simulink model "Calibration_250328"  (R2024b)
settings: Solver=VariableStepAuto  StartTime=0.0  StopTime=Sim.Cal_EndTime  RelTol=1e-3
values from neighbouring files (symbols this model uses):
  m = obj.Br *obj.volume / obj.mu    [External_Magnet2.m]
  Sim = Call_MagneticBasket_Params    [Test.m]    (also in execute_calibrated_result.m; execute_optimized_result.m; optimize_for_calibration.m; optimize_for_max_bending.m)
undefined symbols (not defined in the file or in its folder): X, Y, Z
libraries: sm_lib x64, nesl_utility x43, matrix_library x18, vrlib x12
(part 2 of 2)

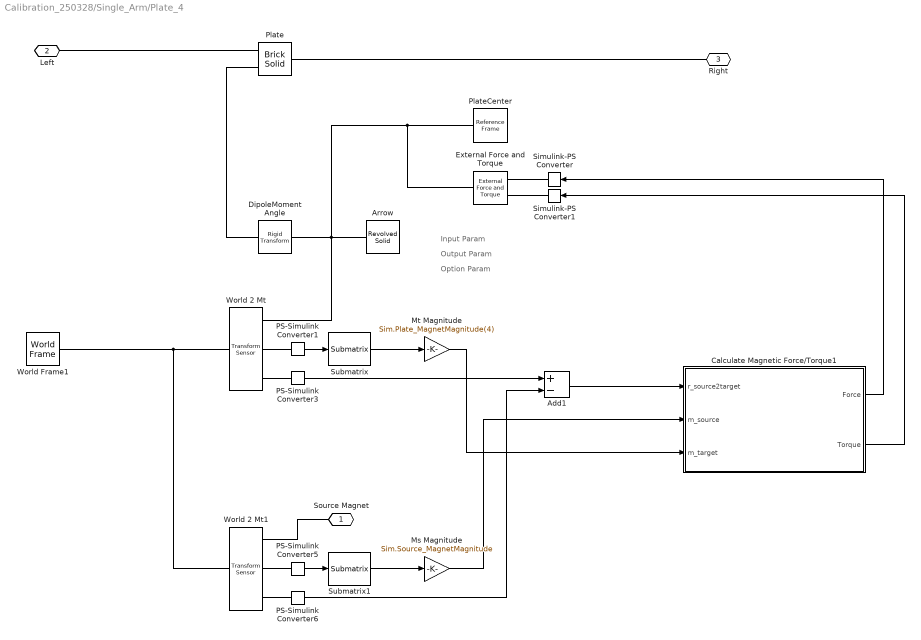
== system Calibration_250328/Single_Arm/Plate_4 ==
  note: Input Param
  note: Output Param
  note: Option Param
  Add1 : Sum  Inputs=+-
  Arrow : sm_lib/Body Elements/Revolved Solid  RevolutionCrossSection=[0 20; 0 0; 1 0; 1 15; 2 15]/10  RevolutionCrossSectionUnits=mm  RevolutionExtent=Full  RevolutionAngle=180  RevolutionAngleUnits=deg  ExportConvexHullGeometry=off  InertiaType=CalculateFromGeometry  BasedOnType=Density  Density=0  DensityUnits=kg/m^3  Mass=1  MassUnits=kg  CenterOfMass=[0 0 0]  CenterOfMassUnits=m  MomentsOfInertia=[1 1 1]  MomentsOfInertiaUnits=kg*m^2  ProductsOfInertia=[0 0 0]  ProductsOfInertiaUnits=kg*m^2  GraphicType=FromGeometry  MarkerShape=Sphere  MarkerSize=10  GraphicVisPropType=SimpleVisualProperties  GraphicDiffuseColor=[0.8 0.0 0.0]  GraphicOpacity=1  GraphicSpecularColor=[0.5 0.5 0.5 1.0]  GraphicAmbientColor=[0.15 0.15 0.15 1.0]  GraphicEmissiveColor=[0.0 0.0 0.0 1.0]  GraphicShininess=75  DoExposeReferenceFrame=on  SerializedFrames=<Frames/>
  Calculate Magnetic Force/Torque1 : Subsystem  AncestorBlock=Manget_DipoleMomentModel_Library_250306/Calculate Magnetic Force//Torque
  DipoleMoment Angle : sm_lib/Frames and Transforms/Rigid Transform  RotationMethod=StandardAxis  FollAlignAxisA=+X  BaseAlignAxisA=+Y  FollAlignAxisB=+Y  BaseAlignAxisB=+Z  RotationStandardAxis=+X  RotationAngle=Sim.Angle(4)  RotationAngleUnits=rad  RotationArbitraryAxis=[0 0 1]  RotationSequenceAxes=FollowerAxes  RotationSequence=XYX  RotationSequenceAngles=[0 0 0]  RotationSequenceAnglesUnits=deg  RotationMatrix=[1 0 0; 0 1 0; 0 0 1]  Quaternion=[1 0 0 0]  TranslationMethod=None  TranslationCartesianOffset=[0 0 0]  TranslationCartesianOffsetUnits=m  TranslationStandardAxis=+Z  TranslationStandardOffset=0  TranslationStandardOffsetUnits=m  TranslationROffset=0  TranslationROffsetUnits=m  TranslationThetaOffset=0  TranslationThetaOffsetUnits=deg  TranslationZOffset=0  TranslationZOffsetUnits=m
  External Force and Torque : sm_lib/Forces and Torques/External Force and Torque  EnableForceX=off  EnableForceY=off  EnableForceZ=off  EnableForce=on  ForceResolutionFrame=World  EnableTorqueX=off  EnableTorqueY=off  EnableTorqueZ=off  EnableTorque=on  TorqueResolutionFrame=World
  Ms Magnitude : Gain  Gain=Sim.Source_MagnetMagnitude
  Mt Magnitude : Gain  Gain=Sim.Plate_MagnetMagnitude(4)
  PS-Simulink Converter{1,3,5..6} (4 alike) : nesl_utility/PS-Simulink Converter  PhysicalDomain=network_engine_domain  SubClassName=ps_output  LeftPortType=input  RightPortType=output  PseudoPeriodic=off  Frequencies=[]  VectorFormat=inherit  Unit=inherit  AffineConversion=off
  Plate : sm_lib/Body Elements/Brick Solid  BrickDimensions=[Sim.PlateWidth Sim.PlateLength Sim.PlateThickness]  BrickDimensionsUnits=m  ExportEntireGeometry=off  InertiaType=CalculateFromGeometry  BasedOnType=Density  Density=Sim.PlateDensity  DensityUnits=kg/m^3  Mass=1  MassUnits=kg  CenterOfMass=[0 0 0]  CenterOfMassUnits=m  MomentsOfInertia=[1 1 1]  MomentsOfInertiaUnits=kg*m^2  ProductsOfInertia=[0 0 0]  ProductsOfInertiaUnits=kg*m^2  GraphicType=FromGeometry  MarkerShape=Sphere  MarkerSize=10  GraphicVisPropType=SimpleVisualProperties  GraphicDiffuseColor=[0.5 0.5 0.5]  GraphicOpacity=0.5  GraphicSpecularColor=[0.5 0.5 0.5 1.0]  GraphicAmbientColor=[0.15 0.15 0.15 1.0]  GraphicEmissiveColor=[0.0 0.0 0.0 1.0]  GraphicShininess=75  DoExposeReferenceFrame=off  SerializedFrames=<Frames><Frame><Id>Frame1</Id><Value><Name>F1</Name><Origin><Source>GeometricFeature</Source><FeatureName>-y -z curve</FeatureName></Origin><PrimaryAxis><DefinedDirection>+Z</DefinedDirection><Source>ReferenceFrame</Source><SourceDirection>+X</SourceDirection><FeatureName></FeatureName></PrimaryAxis><SecondaryAxis><DefinedDirection>+X</DefinedDirection><Source>ReferenceFrame</Source><SourceDirection>+Y</SourceDirection><FeatureName></FeatureName></SecondaryAxis></Value></Frame><Frame><Id>Frame2</Id><Value><Name>F2</Name><Origin><Source>GeometricFeature</Source><FeatureName>+y -z curve</FeatureName></Origin><PrimaryAxis><DefinedDirection>+Z</DefinedDirection><Source>ReferenceFrame</Source><SourceDirection>+X</SourceDirection><FeatureName></FeatureName></PrimaryAxis><SecondaryAxis><DefinedDirection>+X</DefinedDirection><Source>ReferenceFrame</Source><SourceDirection>+Y</SourceDirection><FeatureName></FeatureName></SecondaryAxis></Value></Frame><Frame><Id>Frame3</Id><Value><Name>F3</Name><Origin><Source>ReferenceFrame</Source><FeatureName></FeatureName></Origin><PrimaryAxis><DefinedDirection>+Z</DefinedDirection><Source>ReferenceFrame</Source><SourceDirection>+Y</SourceDirection><FeatureName></FeatureName></PrimaryAxis><SecondaryAxis><DefinedDirection>+X</DefinedDirection><Source>ReferenceFrame</Source><SourceDirection>+X</SourceDirection><FeatureName></FeatureName></SecondaryAxis></Value></Frame></Frames>
  PlateCenter : sm_lib/Frames and Transforms/Reference Frame
  Simulink-PS Converter : nesl_utility/Simulink-PS Converter  PhysicalDomain=network_engine_domain  SubClassName=ps_input  LeftPortType=input  RightPortType=output  PseudoPeriodic=off  Frequencies=[]  NoiseDistribution=none  NoiseParameters=[]  Unit=1  AffineConversion=off  FilteringAndDerivatives=filter  SimscapeFilterOrder=2  InputFilterTimeConstant=0.001  UdotUserProvided=0
  Simulink-PS Converter1 : nesl_utility/Simulink-PS Converter  PhysicalDomain=network_engine_domain  SubClassName=ps_input  LeftPortType=input  RightPortType=output  PseudoPeriodic=off  Frequencies=[]  NoiseDistribution=none  NoiseParameters=[]  Unit=1  AffineConversion=off  FilteringAndDerivatives=filter  SimscapeFilterOrder=2  InputFilterTimeConstant=0.001  UdotUserProvided=0
  Submatrix : matrix_library/Submatrix  RowSpan=All rows  RowStartMode=First  RowStartIndex=1  RowEndMode=Last  RowEndIndex=1  ColSpan=One column  ColStartMode=Last  ColStartIndex=1  ColEndMode=Last  ColEndIndex=1
  Submatrix1 : matrix_library/Submatrix  RowSpan=All rows  RowStartMode=First  RowStartIndex=1  RowEndMode=Last  RowEndIndex=1  ColSpan=One column  ColStartMode=Last  ColStartIndex=1  ColEndMode=Last  ColEndIndex=1
  World 2 Mt : sm_lib/Frames and Transforms/Transform Sensor  MeasurementFrame=World  RotationSequence=XYX  SenseAngle=off  SenseAxis=off  SenseQ=off  SenseR=on  SenseRotationSequence=off  SenseOmegaX=off  SenseOmegaY=off  SenseOmegaZ=off  SenseOmega=off  SenseQDot=off  SenseRDot=off  SenseRotationSequenceDot=off  SenseAlphaX=off  SenseAlphaY=off  SenseAlphaZ=off  SenseAlpha=off  SenseQDDot=off  SenseRDDot=off  SenseX=off  SenseY=off  SenseZ=off  SenseXYZ=on  SenseRad=off  SenseAzim=off  SenseDist=off  SenseInc=off  SenseXDot=off  SenseYDot=off  SenseZDot=off  SenseXYZDot=off  SenseRadDot=off  SenseAzimDot=off  SenseDistDot=off  SenseIncDot=off  SenseXDDot=off  SenseYDDot=off  SenseZDDot=off  SenseXYZDDot=off  SenseRadDDot=off  SenseAzimDDot=off  SenseDistDDot=off  SenseIncDDot=off
  World 2 Mt1 : sm_lib/Frames and Transforms/Transform Sensor  MeasurementFrame=World  RotationSequence=XYX  SenseAngle=off  SenseAxis=off  SenseQ=off  SenseR=on  SenseRotationSequence=off  SenseOmegaX=off  SenseOmegaY=off  SenseOmegaZ=off  SenseOmega=off  SenseQDot=off  SenseRDot=off  SenseRotationSequenceDot=off  SenseAlphaX=off  SenseAlphaY=off  SenseAlphaZ=off  SenseAlpha=off  SenseQDDot=off  SenseRDDot=off  SenseX=off  SenseY=off  SenseZ=off  SenseXYZ=on  SenseRad=off  SenseAzim=off  SenseDist=off  SenseInc=off  SenseXDot=off  SenseYDot=off  SenseZDot=off  SenseXYZDot=off  SenseRadDot=off  SenseAzimDot=off  SenseDistDot=off  SenseIncDot=off  SenseXDDot=off  SenseYDDot=off  SenseZDDot=off  SenseXYZDDot=off  SenseRadDDot=off  SenseAzimDDot=off  SenseDistDDot=off  SenseIncDDot=off
  World Frame1 : sm_lib/Frames and Transforms/World Frame
  Source Magnet : PMIOPort  Side=Left
  Left : PMIOPort  Port=2  Side=Left
  Right : PMIOPort  Port=3  Side=Right
  wires:
  Calculate Magnetic Force/Torque1/2(Torque) -> Simulink-PS Converter1/1
  Calculate Magnetic Force/Torque1/1(Force) -> Simulink-PS Converter/1
  Ms Magnitude/1 -> Calculate Magnetic Force/Torque1/2(m_source)
  Add1/1 -> Calculate Magnetic Force/Torque1/1(r_source2target)
  PS-Simulink Converter6/1 -> Add1/2
  PS-Simulink Converter3/1 -> Add1/1
  Submatrix1/1 -> Ms Magnitude/1
  PS-Simulink Converter5/1 -> Submatrix1/1
  PS-Simulink Converter1/1 -> Submatrix/1
  Mt Magnitude/1 -> Calculate Magnetic Force/Torque1/3(m_target)
  Submatrix/1 -> Mt Magnitude/1
  connections:
  Simulink-PS Converter1/RConn1 -- External Force and Torque/LConn2
  PS-Simulink Converter6/LConn1 -- World 2 Mt1/RConn3
  PS-Simulink Converter5/LConn1 -- World 2 Mt1/RConn2
  Source Magnet/RConn1 -- World 2 Mt1/RConn1
  PS-Simulink Converter3/LConn1 -- World 2 Mt/RConn3
  Plate/LConn2 -- DipoleMoment Angle/LConn1
  World 2 Mt/RConn1 -- DipoleMoment Angle/RConn1 -- Arrow/RConn1 -- External Force and Torque/RConn1 -- PlateCenter/RConn1
  PS-Simulink Converter1/LConn1 -- World 2 Mt/RConn2
  Plate/RConn1 -- Right/RConn1
  World 2 Mt1/LConn1 -- World 2 Mt/LConn1 -- World Frame1/RConn1
  Simulink-PS Converter/RConn1 -- External Force and Torque/LConn1
  Plate/LConn1 -- Left/RConn1

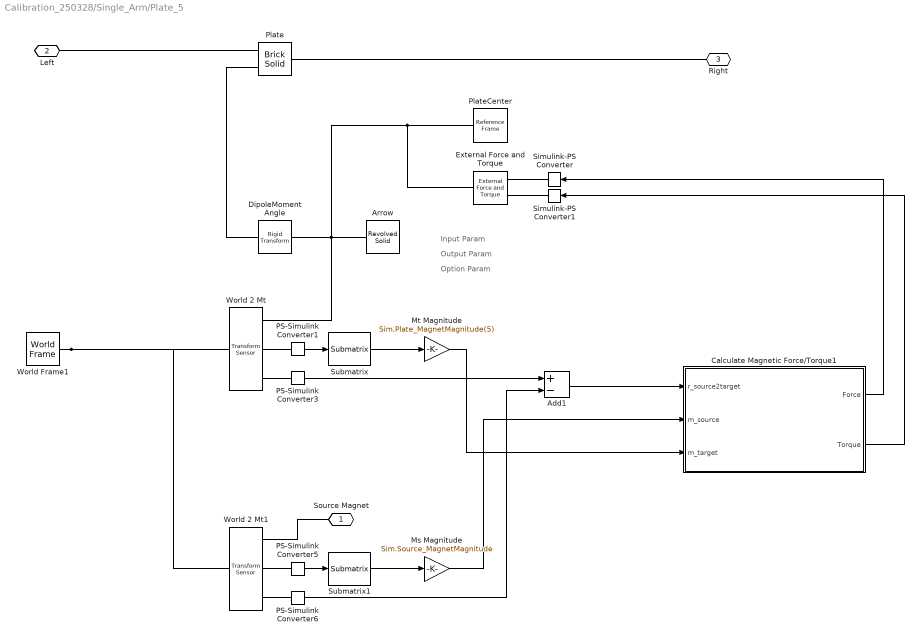
== system Calibration_250328/Single_Arm/Plate_5 ==
  note: Option Param
  note: Output Param
  note: Input Param
  Add1 : Sum  Inputs=+-
  Arrow : sm_lib/Body Elements/Revolved Solid  RevolutionCrossSection=[0 20; 0 0; 1 0; 1 15; 2 15]/10  RevolutionCrossSectionUnits=mm  RevolutionExtent=Full  RevolutionAngle=180  RevolutionAngleUnits=deg  ExportConvexHullGeometry=off  InertiaType=CalculateFromGeometry  BasedOnType=Density  Density=0  DensityUnits=kg/m^3  Mass=1  MassUnits=kg  CenterOfMass=[0 0 0]  CenterOfMassUnits=m  MomentsOfInertia=[1 1 1]  MomentsOfInertiaUnits=kg*m^2  ProductsOfInertia=[0 0 0]  ProductsOfInertiaUnits=kg*m^2  GraphicType=FromGeometry  MarkerShape=Sphere  MarkerSize=10  GraphicVisPropType=SimpleVisualProperties  GraphicDiffuseColor=[0.8 0.0 0.0]  GraphicOpacity=1  GraphicSpecularColor=[0.5 0.5 0.5 1.0]  GraphicAmbientColor=[0.15 0.15 0.15 1.0]  GraphicEmissiveColor=[0.0 0.0 0.0 1.0]  GraphicShininess=75  DoExposeReferenceFrame=on  SerializedFrames=<Frames/>
  Calculate Magnetic Force/Torque1 : Subsystem  AncestorBlock=Manget_DipoleMomentModel_Library_250306/Calculate Magnetic Force//Torque
  DipoleMoment Angle : sm_lib/Frames and Transforms/Rigid Transform  RotationMethod=StandardAxis  FollAlignAxisA=+X  BaseAlignAxisA=+Y  FollAlignAxisB=+Y  BaseAlignAxisB=+Z  RotationStandardAxis=+X  RotationAngle=Sim.Angle(5)  RotationAngleUnits=rad  RotationArbitraryAxis=[0 0 1]  RotationSequenceAxes=FollowerAxes  RotationSequence=XYX  RotationSequenceAngles=[0 0 0]  RotationSequenceAnglesUnits=deg  RotationMatrix=[1 0 0; 0 1 0; 0 0 1]  Quaternion=[1 0 0 0]  TranslationMethod=None  TranslationCartesianOffset=[0 0 0]  TranslationCartesianOffsetUnits=m  TranslationStandardAxis=+Z  TranslationStandardOffset=0  TranslationStandardOffsetUnits=m  TranslationROffset=0  TranslationROffsetUnits=m  TranslationThetaOffset=0  TranslationThetaOffsetUnits=deg  TranslationZOffset=0  TranslationZOffsetUnits=m
  External Force and Torque : sm_lib/Forces and Torques/External Force and Torque  EnableForceX=off  EnableForceY=off  EnableForceZ=off  EnableForce=on  ForceResolutionFrame=World  EnableTorqueX=off  EnableTorqueY=off  EnableTorqueZ=off  EnableTorque=on  TorqueResolutionFrame=World
  Ms Magnitude : Gain  Gain=Sim.Source_MagnetMagnitude
  Mt Magnitude : Gain  Gain=Sim.Plate_MagnetMagnitude(5)
  PS-Simulink Converter{1,3,5..6} (4 alike) : nesl_utility/PS-Simulink Converter  PhysicalDomain=network_engine_domain  SubClassName=ps_output  LeftPortType=input  RightPortType=output  PseudoPeriodic=off  Frequencies=[]  VectorFormat=inherit  Unit=inherit  AffineConversion=off
  Plate : sm_lib/Body Elements/Brick Solid  BrickDimensions=[Sim.PlateWidth Sim.PlateLength Sim.PlateThickness]  BrickDimensionsUnits=m  ExportEntireGeometry=off  InertiaType=CalculateFromGeometry  BasedOnType=Density  Density=Sim.PlateDensity  DensityUnits=kg/m^3  Mass=1  MassUnits=kg  CenterOfMass=[0 0 0]  CenterOfMassUnits=m  MomentsOfInertia=[1 1 1]  MomentsOfInertiaUnits=kg*m^2  ProductsOfInertia=[0 0 0]  ProductsOfInertiaUnits=kg*m^2  GraphicType=FromGeometry  MarkerShape=Sphere  MarkerSize=10  GraphicVisPropType=SimpleVisualProperties  GraphicDiffuseColor=[0.5 0.5 0.5]  GraphicOpacity=0.5  GraphicSpecularColor=[0.5 0.5 0.5 1.0]  GraphicAmbientColor=[0.15 0.15 0.15 1.0]  GraphicEmissiveColor=[0.0 0.0 0.0 1.0]  GraphicShininess=75  DoExposeReferenceFrame=off  SerializedFrames=<Frames><Frame><Id>Frame1</Id><Value><Name>F1</Name><Origin><Source>GeometricFeature</Source><FeatureName>-y -z curve</FeatureName></Origin><PrimaryAxis><DefinedDirection>+Z</DefinedDirection><Source>ReferenceFrame</Source><SourceDirection>+X</SourceDirection><FeatureName></FeatureName></PrimaryAxis><SecondaryAxis><DefinedDirection>+X</DefinedDirection><Source>ReferenceFrame</Source><SourceDirection>+Y</SourceDirection><FeatureName></FeatureName></SecondaryAxis></Value></Frame><Frame><Id>Frame2</Id><Value><Name>F2</Name><Origin><Source>GeometricFeature</Source><FeatureName>+y -z curve</FeatureName></Origin><PrimaryAxis><DefinedDirection>+Z</DefinedDirection><Source>ReferenceFrame</Source><SourceDirection>+X</SourceDirection><FeatureName></FeatureName></PrimaryAxis><SecondaryAxis><DefinedDirection>+X</DefinedDirection><Source>ReferenceFrame</Source><SourceDirection>+Y</SourceDirection><FeatureName></FeatureName></SecondaryAxis></Value></Frame><Frame><Id>Frame3</Id><Value><Name>F3</Name><Origin><Source>ReferenceFrame</Source><FeatureName></FeatureName></Origin><PrimaryAxis><DefinedDirection>+Z</DefinedDirection><Source>ReferenceFrame</Source><SourceDirection>+Y</SourceDirection><FeatureName></FeatureName></PrimaryAxis><SecondaryAxis><DefinedDirection>+X</DefinedDirection><Source>ReferenceFrame</Source><SourceDirection>+X</SourceDirection><FeatureName></FeatureName></SecondaryAxis></Value></Frame></Frames>
  PlateCenter : sm_lib/Frames and Transforms/Reference Frame
  Simulink-PS Converter : nesl_utility/Simulink-PS Converter  PhysicalDomain=network_engine_domain  SubClassName=ps_input  LeftPortType=input  RightPortType=output  PseudoPeriodic=off  Frequencies=[]  NoiseDistribution=none  NoiseParameters=[]  Unit=1  AffineConversion=off  FilteringAndDerivatives=filter  SimscapeFilterOrder=2  InputFilterTimeConstant=0.001  UdotUserProvided=0
  Simulink-PS Converter1 : nesl_utility/Simulink-PS Converter  PhysicalDomain=network_engine_domain  SubClassName=ps_input  LeftPortType=input  RightPortType=output  PseudoPeriodic=off  Frequencies=[]  NoiseDistribution=none  NoiseParameters=[]  Unit=1  AffineConversion=off  FilteringAndDerivatives=filter  SimscapeFilterOrder=2  InputFilterTimeConstant=0.001  UdotUserProvided=0
  Submatrix : matrix_library/Submatrix  RowSpan=All rows  RowStartMode=First  RowStartIndex=1  RowEndMode=Last  RowEndIndex=1  ColSpan=One column  ColStartMode=Last  ColStartIndex=1  ColEndMode=Last  ColEndIndex=1
  Submatrix1 : matrix_library/Submatrix  RowSpan=All rows  RowStartMode=First  RowStartIndex=1  RowEndMode=Last  RowEndIndex=1  ColSpan=One column  ColStartMode=Last  ColStartIndex=1  ColEndMode=Last  ColEndIndex=1
  World 2 Mt : sm_lib/Frames and Transforms/Transform Sensor  MeasurementFrame=World  RotationSequence=XYX  SenseAngle=off  SenseAxis=off  SenseQ=off  SenseR=on  SenseRotationSequence=off  SenseOmegaX=off  SenseOmegaY=off  SenseOmegaZ=off  SenseOmega=off  SenseQDot=off  SenseRDot=off  SenseRotationSequenceDot=off  SenseAlphaX=off  SenseAlphaY=off  SenseAlphaZ=off  SenseAlpha=off  SenseQDDot=off  SenseRDDot=off  SenseX=off  SenseY=off  SenseZ=off  SenseXYZ=on  SenseRad=off  SenseAzim=off  SenseDist=off  SenseInc=off  SenseXDot=off  SenseYDot=off  SenseZDot=off  SenseXYZDot=off  SenseRadDot=off  SenseAzimDot=off  SenseDistDot=off  SenseIncDot=off  SenseXDDot=off  SenseYDDot=off  SenseZDDot=off  SenseXYZDDot=off  SenseRadDDot=off  SenseAzimDDot=off  SenseDistDDot=off  SenseIncDDot=off
  World 2 Mt1 : sm_lib/Frames and Transforms/Transform Sensor  MeasurementFrame=World  RotationSequence=XYX  SenseAngle=off  SenseAxis=off  SenseQ=off  SenseR=on  SenseRotationSequence=off  SenseOmegaX=off  SenseOmegaY=off  SenseOmegaZ=off  SenseOmega=off  SenseQDot=off  SenseRDot=off  SenseRotationSequenceDot=off  SenseAlphaX=off  SenseAlphaY=off  SenseAlphaZ=off  SenseAlpha=off  SenseQDDot=off  SenseRDDot=off  SenseX=off  SenseY=off  SenseZ=off  SenseXYZ=on  SenseRad=off  SenseAzim=off  SenseDist=off  SenseInc=off  SenseXDot=off  SenseYDot=off  SenseZDot=off  SenseXYZDot=off  SenseRadDot=off  SenseAzimDot=off  SenseDistDot=off  SenseIncDot=off  SenseXDDot=off  SenseYDDot=off  SenseZDDot=off  SenseXYZDDot=off  SenseRadDDot=off  SenseAzimDDot=off  SenseDistDDot=off  SenseIncDDot=off
  World Frame1 : sm_lib/Frames and Transforms/World Frame
  Source Magnet : PMIOPort  Side=Left
  Left : PMIOPort  Port=2  Side=Left
  Right : PMIOPort  Port=3  Side=Right
  wires:
  Submatrix/1 -> Mt Magnitude/1
  Mt Magnitude/1 -> Calculate Magnetic Force/Torque1/3(m_target)
  PS-Simulink Converter1/1 -> Submatrix/1
  PS-Simulink Converter5/1 -> Submatrix1/1
  Submatrix1/1 -> Ms Magnitude/1
  PS-Simulink Converter3/1 -> Add1/1
  PS-Simulink Converter6/1 -> Add1/2
  Add1/1 -> Calculate Magnetic Force/Torque1/1(r_source2target)
  Ms Magnitude/1 -> Calculate Magnetic Force/Torque1/2(m_source)
  Calculate Magnetic Force/Torque1/1(Force) -> Simulink-PS Converter/1
  Calculate Magnetic Force/Torque1/2(Torque) -> Simulink-PS Converter1/1
  connections:
  Plate/LConn1 -- Left/RConn1
  Simulink-PS Converter/RConn1 -- External Force and Torque/LConn1
  World Frame1/RConn1 -- World 2 Mt/LConn1 -- World 2 Mt1/LConn1
  Plate/RConn1 -- Right/RConn1
  PS-Simulink Converter1/LConn1 -- World 2 Mt/RConn2
  PlateCenter/RConn1 -- External Force and Torque/RConn1 -- Arrow/RConn1 -- DipoleMoment Angle/RConn1 -- World 2 Mt/RConn1
  Plate/LConn2 -- DipoleMoment Angle/LConn1
  PS-Simulink Converter3/LConn1 -- World 2 Mt/RConn3
  Source Magnet/RConn1 -- World 2 Mt1/RConn1
  PS-Simulink Converter5/LConn1 -- World 2 Mt1/RConn2
  PS-Simulink Converter6/LConn1 -- World 2 Mt1/RConn3
  Simulink-PS Converter1/RConn1 -- External Force and Torque/LConn2

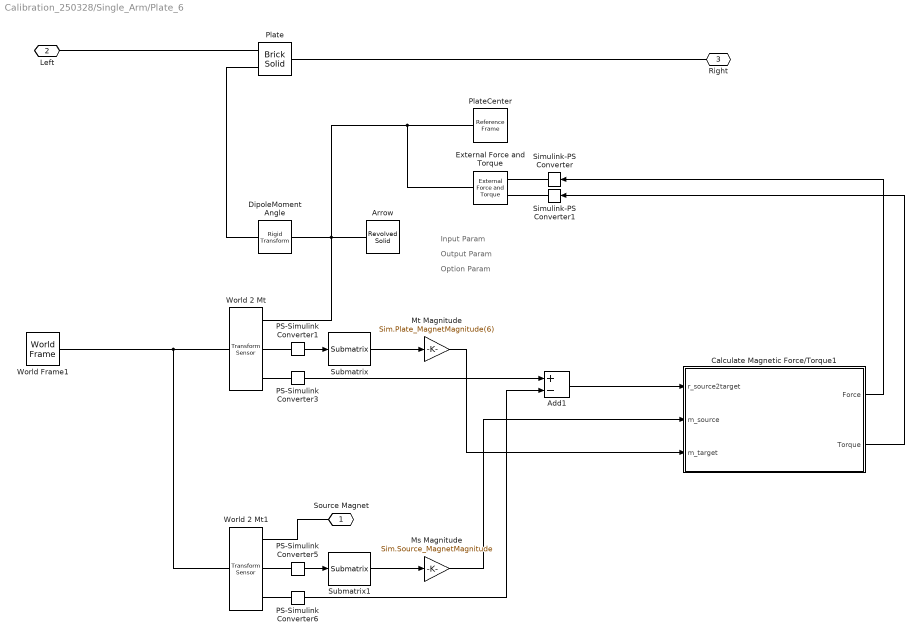
== system Calibration_250328/Single_Arm/Plate_6 ==
  note: Input Param
  note: Output Param
  note: Option Param
  Add1 : Sum  Inputs=+-
  Arrow : sm_lib/Body Elements/Revolved Solid  RevolutionCrossSection=[0 20; 0 0; 1 0; 1 15; 2 15]/10  RevolutionCrossSectionUnits=mm  RevolutionExtent=Full  RevolutionAngle=180  RevolutionAngleUnits=deg  ExportConvexHullGeometry=off  InertiaType=CalculateFromGeometry  BasedOnType=Density  Density=0  DensityUnits=kg/m^3  Mass=1  MassUnits=kg  CenterOfMass=[0 0 0]  CenterOfMassUnits=m  MomentsOfInertia=[1 1 1]  MomentsOfInertiaUnits=kg*m^2  ProductsOfInertia=[0 0 0]  ProductsOfInertiaUnits=kg*m^2  GraphicType=FromGeometry  MarkerShape=Sphere  MarkerSize=10  GraphicVisPropType=SimpleVisualProperties  GraphicDiffuseColor=[0.8 0.0 0.0]  GraphicOpacity=1  GraphicSpecularColor=[0.5 0.5 0.5 1.0]  GraphicAmbientColor=[0.15 0.15 0.15 1.0]  GraphicEmissiveColor=[0.0 0.0 0.0 1.0]  GraphicShininess=75  DoExposeReferenceFrame=on  SerializedFrames=<Frames/>
  Calculate Magnetic Force/Torque1 : Subsystem  AncestorBlock=Manget_DipoleMomentModel_Library_250306/Calculate Magnetic Force//Torque
  DipoleMoment Angle : sm_lib/Frames and Transforms/Rigid Transform  RotationMethod=StandardAxis  FollAlignAxisA=+X  BaseAlignAxisA=+Y  FollAlignAxisB=+Y  BaseAlignAxisB=+Z  RotationStandardAxis=+X  RotationAngle=Sim.Angle(6)  RotationAngleUnits=rad  RotationArbitraryAxis=[0 0 1]  RotationSequenceAxes=FollowerAxes  RotationSequence=XYX  RotationSequenceAngles=[0 0 0]  RotationSequenceAnglesUnits=deg  RotationMatrix=[1 0 0; 0 1 0; 0 0 1]  Quaternion=[1 0 0 0]  TranslationMethod=None  TranslationCartesianOffset=[0 0 0]  TranslationCartesianOffsetUnits=m  TranslationStandardAxis=+Z  TranslationStandardOffset=0  TranslationStandardOffsetUnits=m  TranslationROffset=0  TranslationROffsetUnits=m  TranslationThetaOffset=0  TranslationThetaOffsetUnits=deg  TranslationZOffset=0  TranslationZOffsetUnits=m
  External Force and Torque : sm_lib/Forces and Torques/External Force and Torque  EnableForceX=off  EnableForceY=off  EnableForceZ=off  EnableForce=on  ForceResolutionFrame=World  EnableTorqueX=off  EnableTorqueY=off  EnableTorqueZ=off  EnableTorque=on  TorqueResolutionFrame=World
  Ms Magnitude : Gain  Gain=Sim.Source_MagnetMagnitude
  Mt Magnitude : Gain  Gain=Sim.Plate_MagnetMagnitude(6)
  PS-Simulink Converter{1,3,5..6} (4 alike) : nesl_utility/PS-Simulink Converter  PhysicalDomain=network_engine_domain  SubClassName=ps_output  LeftPortType=input  RightPortType=output  PseudoPeriodic=off  Frequencies=[]  VectorFormat=inherit  Unit=inherit  AffineConversion=off
  Plate : sm_lib/Body Elements/Brick Solid  BrickDimensions=[Sim.PlateWidth Sim.PlateLength Sim.PlateThickness]  BrickDimensionsUnits=m  ExportEntireGeometry=off  InertiaType=CalculateFromGeometry  BasedOnType=Density  Density=Sim.PlateDensity  DensityUnits=kg/m^3  Mass=1  MassUnits=kg  CenterOfMass=[0 0 0]  CenterOfMassUnits=m  MomentsOfInertia=[1 1 1]  MomentsOfInertiaUnits=kg*m^2  ProductsOfInertia=[0 0 0]  ProductsOfInertiaUnits=kg*m^2  GraphicType=FromGeometry  MarkerShape=Sphere  MarkerSize=10  GraphicVisPropType=SimpleVisualProperties  GraphicDiffuseColor=[0.5 0.5 0.5]  GraphicOpacity=0.5  GraphicSpecularColor=[0.5 0.5 0.5 1.0]  GraphicAmbientColor=[0.15 0.15 0.15 1.0]  GraphicEmissiveColor=[0.0 0.0 0.0 1.0]  GraphicShininess=75  DoExposeReferenceFrame=off  SerializedFrames=<Frames><Frame><Id>Frame1</Id><Value><Name>F1</Name><Origin><Source>GeometricFeature</Source><FeatureName>-y -z curve</FeatureName></Origin><PrimaryAxis><DefinedDirection>+Z</DefinedDirection><Source>ReferenceFrame</Source><SourceDirection>+X</SourceDirection><FeatureName></FeatureName></PrimaryAxis><SecondaryAxis><DefinedDirection>+X</DefinedDirection><Source>ReferenceFrame</Source><SourceDirection>+Y</SourceDirection><FeatureName></FeatureName></SecondaryAxis></Value></Frame><Frame><Id>Frame2</Id><Value><Name>F2</Name><Origin><Source>GeometricFeature</Source><FeatureName>+y -z curve</FeatureName></Origin><PrimaryAxis><DefinedDirection>+Z</DefinedDirection><Source>ReferenceFrame</Source><SourceDirection>+X</SourceDirection><FeatureName></FeatureName></PrimaryAxis><SecondaryAxis><DefinedDirection>+X</DefinedDirection><Source>ReferenceFrame</Source><SourceDirection>+Y</SourceDirection><FeatureName></FeatureName></SecondaryAxis></Value></Frame><Frame><Id>Frame3</Id><Value><Name>F3</Name><Origin><Source>ReferenceFrame</Source><FeatureName></FeatureName></Origin><PrimaryAxis><DefinedDirection>+Z</DefinedDirection><Source>ReferenceFrame</Source><SourceDirection>+Y</SourceDirection><FeatureName></FeatureName></PrimaryAxis><SecondaryAxis><DefinedDirection>+X</DefinedDirection><Source>ReferenceFrame</Source><SourceDirection>+X</SourceDirection><FeatureName></FeatureName></SecondaryAxis></Value></Frame></Frames>
  PlateCenter : sm_lib/Frames and Transforms/Reference Frame
  Simulink-PS Converter : nesl_utility/Simulink-PS Converter  PhysicalDomain=network_engine_domain  SubClassName=ps_input  LeftPortType=input  RightPortType=output  PseudoPeriodic=off  Frequencies=[]  NoiseDistribution=none  NoiseParameters=[]  Unit=1  AffineConversion=off  FilteringAndDerivatives=filter  SimscapeFilterOrder=2  InputFilterTimeConstant=0.001  UdotUserProvided=0
  Simulink-PS Converter1 : nesl_utility/Simulink-PS Converter  PhysicalDomain=network_engine_domain  SubClassName=ps_input  LeftPortType=input  RightPortType=output  PseudoPeriodic=off  Frequencies=[]  NoiseDistribution=none  NoiseParameters=[]  Unit=1  AffineConversion=off  FilteringAndDerivatives=filter  SimscapeFilterOrder=2  InputFilterTimeConstant=0.001  UdotUserProvided=0
  Submatrix : matrix_library/Submatrix  RowSpan=All rows  RowStartMode=First  RowStartIndex=1  RowEndMode=Last  RowEndIndex=1  ColSpan=One column  ColStartMode=Last  ColStartIndex=1  ColEndMode=Last  ColEndIndex=1
  Submatrix1 : matrix_library/Submatrix  RowSpan=All rows  RowStartMode=First  RowStartIndex=1  RowEndMode=Last  RowEndIndex=1  ColSpan=One column  ColStartMode=Last  ColStartIndex=1  ColEndMode=Last  ColEndIndex=1
  World 2 Mt : sm_lib/Frames and Transforms/Transform Sensor  MeasurementFrame=World  RotationSequence=XYX  SenseAngle=off  SenseAxis=off  SenseQ=off  SenseR=on  SenseRotationSequence=off  SenseOmegaX=off  SenseOmegaY=off  SenseOmegaZ=off  SenseOmega=off  SenseQDot=off  SenseRDot=off  SenseRotationSequenceDot=off  SenseAlphaX=off  SenseAlphaY=off  SenseAlphaZ=off  SenseAlpha=off  SenseQDDot=off  SenseRDDot=off  SenseX=off  SenseY=off  SenseZ=off  SenseXYZ=on  SenseRad=off  SenseAzim=off  SenseDist=off  SenseInc=off  SenseXDot=off  SenseYDot=off  SenseZDot=off  SenseXYZDot=off  SenseRadDot=off  SenseAzimDot=off  SenseDistDot=off  SenseIncDot=off  SenseXDDot=off  SenseYDDot=off  SenseZDDot=off  SenseXYZDDot=off  SenseRadDDot=off  SenseAzimDDot=off  SenseDistDDot=off  SenseIncDDot=off
  World 2 Mt1 : sm_lib/Frames and Transforms/Transform Sensor  MeasurementFrame=World  RotationSequence=XYX  SenseAngle=off  SenseAxis=off  SenseQ=off  SenseR=on  SenseRotationSequence=off  SenseOmegaX=off  SenseOmegaY=off  SenseOmegaZ=off  SenseOmega=off  SenseQDot=off  SenseRDot=off  SenseRotationSequenceDot=off  SenseAlphaX=off  SenseAlphaY=off  SenseAlphaZ=off  SenseAlpha=off  SenseQDDot=off  SenseRDDot=off  SenseX=off  SenseY=off  SenseZ=off  SenseXYZ=on  SenseRad=off  SenseAzim=off  SenseDist=off  SenseInc=off  SenseXDot=off  SenseYDot=off  SenseZDot=off  SenseXYZDot=off  SenseRadDot=off  SenseAzimDot=off  SenseDistDot=off  SenseIncDot=off  SenseXDDot=off  SenseYDDot=off  SenseZDDot=off  SenseXYZDDot=off  SenseRadDDot=off  SenseAzimDDot=off  SenseDistDDot=off  SenseIncDDot=off
  World Frame1 : sm_lib/Frames and Transforms/World Frame
  Source Magnet : PMIOPort  Side=Left
  Left : PMIOPort  Port=2  Side=Left
  Right : PMIOPort  Port=3  Side=Right
  wires:
  Calculate Magnetic Force/Torque1/2(Torque) -> Simulink-PS Converter1/1
  Calculate Magnetic Force/Torque1/1(Force) -> Simulink-PS Converter/1
  Ms Magnitude/1 -> Calculate Magnetic Force/Torque1/2(m_source)
  Add1/1 -> Calculate Magnetic Force/Torque1/1(r_source2target)
  PS-Simulink Converter6/1 -> Add1/2
  PS-Simulink Converter3/1 -> Add1/1
  Submatrix1/1 -> Ms Magnitude/1
  PS-Simulink Converter5/1 -> Submatrix1/1
  PS-Simulink Converter1/1 -> Submatrix/1
  Mt Magnitude/1 -> Calculate Magnetic Force/Torque1/3(m_target)
  Submatrix/1 -> Mt Magnitude/1
  connections:
  Simulink-PS Converter1/RConn1 -- External Force and Torque/LConn2
  PS-Simulink Converter6/LConn1 -- World 2 Mt1/RConn3
  PS-Simulink Converter5/LConn1 -- World 2 Mt1/RConn2
  Source Magnet/RConn1 -- World 2 Mt1/RConn1
  PS-Simulink Converter3/LConn1 -- World 2 Mt/RConn3
  Plate/LConn2 -- DipoleMoment Angle/LConn1
  World 2 Mt/RConn1 -- DipoleMoment Angle/RConn1 -- Arrow/RConn1 -- External Force and Torque/RConn1 -- PlateCenter/RConn1
  PS-Simulink Converter1/LConn1 -- World 2 Mt/RConn2
  Plate/RConn1 -- Right/RConn1
  World 2 Mt1/LConn1 -- World 2 Mt/LConn1 -- World Frame1/RConn1
  Simulink-PS Converter/RConn1 -- External Force and Torque/LConn1
  Plate/LConn1 -- Left/RConn1

== system Calibration_250328/Single_Arm/Plate_1/Calculate Magnetic Force//Torque1 ==
  r_source2target : Inport
  m_source : Inport  Port=2
  m_target : Inport  Port=3
  Magnetic Force : Subsystem  AncestorBlock=Manget_DipoleMomentModel_Library_250306/Magnetic Force
  Magnetic Torque : Subsystem  AncestorBlock=Manget_DipoleMomentModel_Library_250306/Magnetic Torque
  Force : Outport
  Torque : Outport  Port=2
  wires:
  m_source/1 -> Magnetic Force/2(m_source), Magnetic Torque/2(m_source)
  m_target/1 -> Magnetic Torque/3(m_target), Magnetic Force/3(m_target)
  r_source2target/1 -> Magnetic Force/1(r_source2target), Magnetic Torque/1(r_source2target)
  Magnetic Torque/1(Torque) -> Torque/1
  Magnetic Force/1(Force) -> Force/1

== system Calibration_250328/Single_Arm/Plate_2/Calculate Magnetic Force//Torque1 ==
  r_source2target : Inport
  m_source : Inport  Port=2
  m_target : Inport  Port=3
  Magnetic Force : Subsystem  AncestorBlock=Manget_DipoleMomentModel_Library_250306/Magnetic Force
  Magnetic Torque : Subsystem  AncestorBlock=Manget_DipoleMomentModel_Library_250306/Magnetic Torque
  Force : Outport
  Torque : Outport  Port=2
  wires:
  Magnetic Force/1(Force) -> Force/1
  Magnetic Torque/1(Torque) -> Torque/1
  r_source2target/1 -> Magnetic Torque/1(r_source2target), Magnetic Force/1(r_source2target)
  m_target/1 -> Magnetic Force/3(m_target), Magnetic Torque/3(m_target)
  m_source/1 -> Magnetic Torque/2(m_source), Magnetic Force/2(m_source)

== system Calibration_250328/Single_Arm/Plate_3/Calculate Magnetic Force//Torque1 ==
  r_source2target : Inport
  m_source : Inport  Port=2
  m_target : Inport  Port=3
  Magnetic Force : Subsystem  AncestorBlock=Manget_DipoleMomentModel_Library_250306/Magnetic Force
  Magnetic Torque : Subsystem  AncestorBlock=Manget_DipoleMomentModel_Library_250306/Magnetic Torque
  Force : Outport
  Torque : Outport  Port=2
  wires:
  m_source/1 -> Magnetic Force/2(m_source), Magnetic Torque/2(m_source)
  m_target/1 -> Magnetic Torque/3(m_target), Magnetic Force/3(m_target)
  r_source2target/1 -> Magnetic Force/1(r_source2target), Magnetic Torque/1(r_source2target)
  Magnetic Torque/1(Torque) -> Torque/1
  Magnetic Force/1(Force) -> Force/1

== system Calibration_250328/Single_Arm/Plate_4/Calculate Magnetic Force//Torque1 ==
  r_source2target : Inport
  m_source : Inport  Port=2
  m_target : Inport  Port=3
  Magnetic Force : Subsystem  AncestorBlock=Manget_DipoleMomentModel_Library_250306/Magnetic Force
  Magnetic Torque : Subsystem  AncestorBlock=Manget_DipoleMomentModel_Library_250306/Magnetic Torque
  Force : Outport
  Torque : Outport  Port=2
  wires:
  Magnetic Force/1(Force) -> Force/1
  Magnetic Torque/1(Torque) -> Torque/1
  r_source2target/1 -> Magnetic Torque/1(r_source2target), Magnetic Force/1(r_source2target)
  m_target/1 -> Magnetic Force/3(m_target), Magnetic Torque/3(m_target)
  m_source/1 -> Magnetic Torque/2(m_source), Magnetic Force/2(m_source)

== system Calibration_250328/Single_Arm/Plate_5/Calculate Magnetic Force//Torque1 ==
  r_source2target : Inport
  m_source : Inport  Port=2
  m_target : Inport  Port=3
  Magnetic Force : Subsystem  AncestorBlock=Manget_DipoleMomentModel_Library_250306/Magnetic Force
  Magnetic Torque : Subsystem  AncestorBlock=Manget_DipoleMomentModel_Library_250306/Magnetic Torque
  Force : Outport
  Torque : Outport  Port=2
  wires:
  m_source/1 -> Magnetic Force/2(m_source), Magnetic Torque/2(m_source)
  m_target/1 -> Magnetic Torque/3(m_target), Magnetic Force/3(m_target)
  r_source2target/1 -> Magnetic Force/1(r_source2target), Magnetic Torque/1(r_source2target)
  Magnetic Torque/1(Torque) -> Torque/1
  Magnetic Force/1(Force) -> Force/1

== system Calibration_250328/Single_Arm/Plate_6/Calculate Magnetic Force//Torque1 ==
  r_source2target : Inport
  m_source : Inport  Port=2
  m_target : Inport  Port=3
  Magnetic Force : Subsystem  AncestorBlock=Manget_DipoleMomentModel_Library_250306/Magnetic Force
  Magnetic Torque : Subsystem  AncestorBlock=Manget_DipoleMomentModel_Library_250306/Magnetic Torque
  Force : Outport
  Torque : Outport  Port=2
  wires:
  Magnetic Force/1(Force) -> Force/1
  Magnetic Torque/1(Torque) -> Torque/1
  r_source2target/1 -> Magnetic Torque/1(r_source2target), Magnetic Force/1(r_source2target)
  m_target/1 -> Magnetic Force/3(m_target), Magnetic Torque/3(m_target)
  m_source/1 -> Magnetic Torque/2(m_source), Magnetic Force/2(m_source)

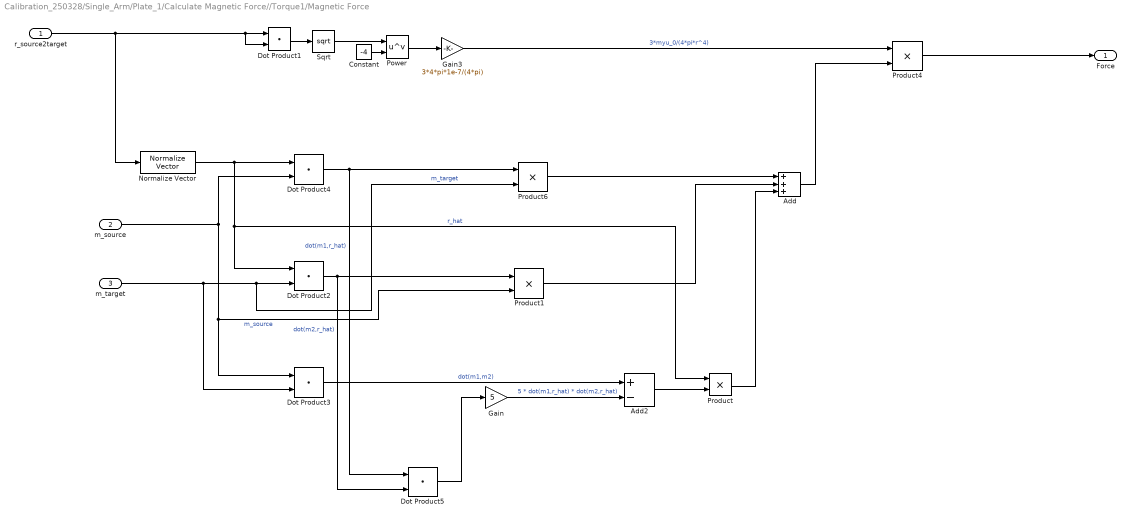
== system Calibration_250328/Single_Arm/Plate_1/Calculate Magnetic Force//Torque1/Magnetic Force ==
  r_source2target : Inport
  m_source : Inport  Port=2
  m_target : Inport  Port=3
  Add : Sum  Inputs=+++
  Add2 : Sum  Inputs=+-
  Constant : Constant  Value=-4
  Dot Product{1..5} (5 alike) : DotProduct  OutDataTypeStr=Inherit: Inherit via internal rule
  Gain : Gain  Gain=5
  Gain3 : Gain  Gain=3*4*pi*1e-7/(4*pi)
  Normalize Vector : vrlib/Utilities/Normalize Vector  maxzero=0
  Power : Math  Operator=pow
  Product{,1,4,6} (4 alike) : Product
  Sqrt : Sqrt
  Force : Outport
  wires:
  Sqrt/1 -> Power/1
  Product/1 -> Add/3
  Add2/1 -> Product/2
  Add/1 -> Product4/2
  Product6/1 -> Add/1
  Product1/1 -> Add/2
  Gain/1 -> Add2/2  "5 * dot(m1,r_hat) * dot(m2,r_hat)"
  Dot Product5/1 -> Gain/1
  Dot Product3/1 -> Add2/1  "dot(m1,m2)"
  Dot Product2/1 -> Dot Product5/2, Product1/1  "dot(m2,r_hat)"
  Dot Product4/1 -> Dot Product5/1, Product6/1  "dot(m1,r_hat)"
  m_target/1 -> Product6/2, Dot Product2/2, Dot Product3/2  "m_target"
  m_source/1 -> Dot Product4/2, Product1/2, Dot Product3/1  "m_source"
  Normalize Vector/1 -> Dot Product4/1, Dot Product2/1, Product/1  "r_hat"
  r_source2target/1 -> Dot Product1/1, Dot Product1/2, Normalize Vector/1
  Product4/1 -> Force/1
  Gain3/1 -> Product4/1  "3*myu_0/(4*pi*r^4)"
  Power/1 -> Gain3/1
  Constant/1 -> Power/2
  Dot Product1/1 -> Sqrt/1

== system Calibration_250328/Single_Arm/Plate_1/Calculate Magnetic Force//Torque1/Magnetic Torque ==
  note: 모든 좌표계는 World Frame 기준!
  r_source2target : Inport
  m_source : Inport  Port=2
  m_target : Inport  Port=3
  Add : Sum  Inputs=+-
  Constant : Constant  Value=-3
  Constant1 : Constant  Value=eye(3)
  Cross Product : matrix_library/Cross Product
  Dot Product : DotProduct  OutDataTypeStr=Inherit: Inherit via internal rule
  Gain : Gain  Gain=4*pi*1e-7/(4*pi)
  Gain1 : Gain  Gain=3
  MatrixMultiply : Product  Multiplication=Matrix(*)
  MatrixMultiply1 : Product  Multiplication=Matrix(*)
  Normalize Vector : vrlib/Utilities/Normalize Vector  maxzero=0
  Power : Math  Operator=pow
  Product : Product
  Sqrt : Sqrt
  Transpose : Math  Operator=transpose
  Torque : Outport
  wires:
  Sqrt/1 -> Power/1
  Gain1/1 -> Add/1
  Product/1 -> Cross Product/2
  MatrixMultiply1/1 -> Product/1
  Gain/1 -> Product/2
  m_source/1 -> MatrixMultiply1/2
  Add/1 -> MatrixMultiply1/1
  Constant1/1 -> Add/2
  MatrixMultiply/1 -> Gain1/1
  Transpose/1 -> MatrixMultiply/2
  Normalize Vector/1 -> MatrixMultiply/1, Transpose/1
  Power/1 -> Gain/1
  Constant/1 -> Power/2
  Dot Product/1 -> Sqrt/1
  r_source2target/1 -> Normalize Vector/1, Dot Product/1, Dot Product/2
  m_target/1 -> Cross Product/1
  Cross Product/1 -> Torque/1

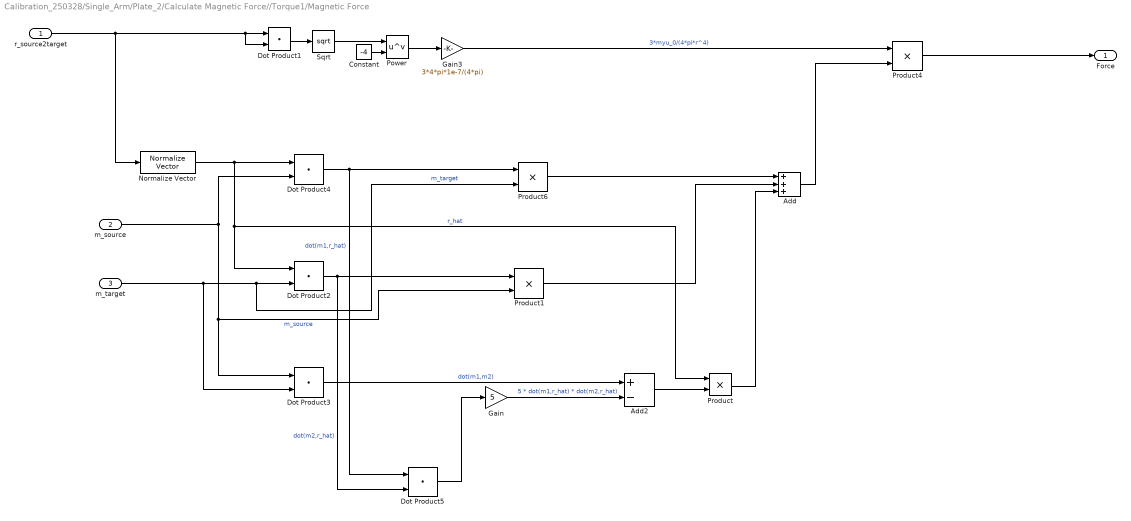
== system Calibration_250328/Single_Arm/Plate_2/Calculate Magnetic Force//Torque1/Magnetic Force ==
  r_source2target : Inport
  m_source : Inport  Port=2
  m_target : Inport  Port=3
  Add : Sum  Inputs=+++
  Add2 : Sum  Inputs=+-
  Constant : Constant  Value=-4
  Dot Product{1..5} (5 alike) : DotProduct  OutDataTypeStr=Inherit: Inherit via internal rule
  Gain : Gain  Gain=5
  Gain3 : Gain  Gain=3*4*pi*1e-7/(4*pi)
  Normalize Vector : vrlib/Utilities/Normalize Vector  maxzero=0
  Power : Math  Operator=pow
  Product{,1,4,6} (4 alike) : Product
  Sqrt : Sqrt
  Force : Outport
  wires:
  Dot Product1/1 -> Sqrt/1
  Constant/1 -> Power/2
  Power/1 -> Gain3/1
  Gain3/1 -> Product4/1  "3*myu_0/(4*pi*r^4)"
  Product4/1 -> Force/1
  r_source2target/1 -> Normalize Vector/1, Dot Product1/2, Dot Product1/1
  Normalize Vector/1 -> Product/1, Dot Product2/1, Dot Product4/1  "r_hat"
  m_source/1 -> Dot Product3/1, Product1/2, Dot Product4/2  "m_source"
  m_target/1 -> Dot Product3/2, Dot Product2/2, Product6/2  "m_target"
  Dot Product4/1 -> Product6/1, Dot Product5/1  "dot(m1,r_hat)"
  Dot Product2/1 -> Product1/1, Dot Product5/2  "dot(m2,r_hat)"
  Dot Product3/1 -> Add2/1  "dot(m1,m2)"
  Dot Product5/1 -> Gain/1
  Gain/1 -> Add2/2  "5 * dot(m1,r_hat) * dot(m2,r_hat)"
  Product1/1 -> Add/2
  Product6/1 -> Add/1
  Add/1 -> Product4/2
  Add2/1 -> Product/2
  Product/1 -> Add/3
  Sqrt/1 -> Power/1

== system Calibration_250328/Single_Arm/Plate_2/Calculate Magnetic Force//Torque1/Magnetic Torque ==
  note: 모든 좌표계는 World Frame 기준!
  r_source2target : Inport
  m_source : Inport  Port=2
  m_target : Inport  Port=3
  Add : Sum  Inputs=+-
  Constant : Constant  Value=-3
  Constant1 : Constant  Value=eye(3)
  Cross Product : matrix_library/Cross Product
  Dot Product : DotProduct  OutDataTypeStr=Inherit: Inherit via internal rule
  Gain : Gain  Gain=4*pi*1e-7/(4*pi)
  Gain1 : Gain  Gain=3
  MatrixMultiply : Product  Multiplication=Matrix(*)
  MatrixMultiply1 : Product  Multiplication=Matrix(*)
  Normalize Vector : vrlib/Utilities/Normalize Vector  maxzero=0
  Power : Math  Operator=pow
  Product : Product
  Sqrt : Sqrt
  Transpose : Math  Operator=transpose
  Torque : Outport
  wires:
  Cross Product/1 -> Torque/1
  m_target/1 -> Cross Product/1
  r_source2target/1 -> Dot Product/2, Dot Product/1, Normalize Vector/1
  Dot Product/1 -> Sqrt/1
  Constant/1 -> Power/2
  Power/1 -> Gain/1
  Normalize Vector/1 -> Transpose/1, MatrixMultiply/1
  Transpose/1 -> MatrixMultiply/2
  MatrixMultiply/1 -> Gain1/1
  Constant1/1 -> Add/2
  Add/1 -> MatrixMultiply1/1
  m_source/1 -> MatrixMultiply1/2
  Gain/1 -> Product/2
  MatrixMultiply1/1 -> Product/1
  Product/1 -> Cross Product/2
  Gain1/1 -> Add/1
  Sqrt/1 -> Power/1

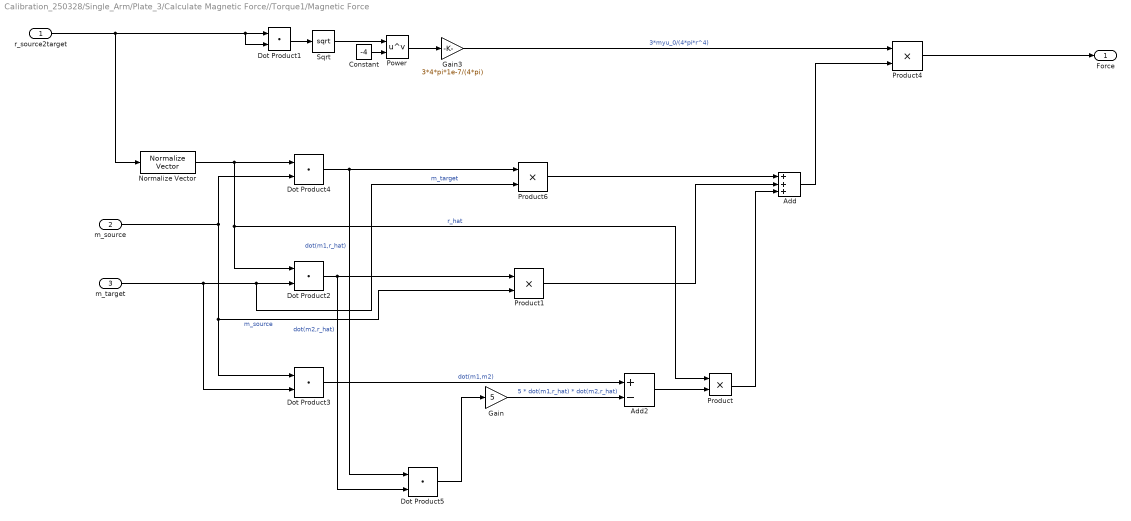
== system Calibration_250328/Single_Arm/Plate_3/Calculate Magnetic Force//Torque1/Magnetic Force ==
  r_source2target : Inport
  m_source : Inport  Port=2
  m_target : Inport  Port=3
  Add : Sum  Inputs=+++
  Add2 : Sum  Inputs=+-
  Constant : Constant  Value=-4
  Dot Product{1..5} (5 alike) : DotProduct  OutDataTypeStr=Inherit: Inherit via internal rule
  Gain : Gain  Gain=5
  Gain3 : Gain  Gain=3*4*pi*1e-7/(4*pi)
  Normalize Vector : vrlib/Utilities/Normalize Vector  maxzero=0
  Power : Math  Operator=pow
  Product{,1,4,6} (4 alike) : Product
  Sqrt : Sqrt
  Force : Outport
  wires:
  Sqrt/1 -> Power/1
  Product/1 -> Add/3
  Add2/1 -> Product/2
  Add/1 -> Product4/2
  Product6/1 -> Add/1
  Product1/1 -> Add/2
  Gain/1 -> Add2/2  "5 * dot(m1,r_hat) * dot(m2,r_hat)"
  Dot Product5/1 -> Gain/1
  Dot Product3/1 -> Add2/1  "dot(m1,m2)"
  Dot Product2/1 -> Dot Product5/2, Product1/1  "dot(m2,r_hat)"
  Dot Product4/1 -> Dot Product5/1, Product6/1  "dot(m1,r_hat)"
  m_target/1 -> Product6/2, Dot Product2/2, Dot Product3/2  "m_target"
  m_source/1 -> Dot Product4/2, Product1/2, Dot Product3/1  "m_source"
  Normalize Vector/1 -> Dot Product4/1, Dot Product2/1, Product/1  "r_hat"
  r_source2target/1 -> Dot Product1/1, Dot Product1/2, Normalize Vector/1
  Product4/1 -> Force/1
  Gain3/1 -> Product4/1  "3*myu_0/(4*pi*r^4)"
  Power/1 -> Gain3/1
  Constant/1 -> Power/2
  Dot Product1/1 -> Sqrt/1

== system Calibration_250328/Single_Arm/Plate_3/Calculate Magnetic Force//Torque1/Magnetic Torque ==
  note: 모든 좌표계는 World Frame 기준!
  r_source2target : Inport
  m_source : Inport  Port=2
  m_target : Inport  Port=3
  Add : Sum  Inputs=+-
  Constant : Constant  Value=-3
  Constant1 : Constant  Value=eye(3)
  Cross Product : matrix_library/Cross Product
  Dot Product : DotProduct  OutDataTypeStr=Inherit: Inherit via internal rule
  Gain : Gain  Gain=4*pi*1e-7/(4*pi)
  Gain1 : Gain  Gain=3
  MatrixMultiply : Product  Multiplication=Matrix(*)
  MatrixMultiply1 : Product  Multiplication=Matrix(*)
  Normalize Vector : vrlib/Utilities/Normalize Vector  maxzero=0
  Power : Math  Operator=pow
  Product : Product
  Sqrt : Sqrt
  Transpose : Math  Operator=transpose
  Torque : Outport
  wires:
  Sqrt/1 -> Power/1
  Gain1/1 -> Add/1
  Product/1 -> Cross Product/2
  MatrixMultiply1/1 -> Product/1
  Gain/1 -> Product/2
  m_source/1 -> MatrixMultiply1/2
  Add/1 -> MatrixMultiply1/1
  Constant1/1 -> Add/2
  MatrixMultiply/1 -> Gain1/1
  Transpose/1 -> MatrixMultiply/2
  Normalize Vector/1 -> MatrixMultiply/1, Transpose/1
  Power/1 -> Gain/1
  Constant/1 -> Power/2
  Dot Product/1 -> Sqrt/1
  r_source2target/1 -> Normalize Vector/1, Dot Product/1, Dot Product/2
  m_target/1 -> Cross Product/1
  Cross Product/1 -> Torque/1

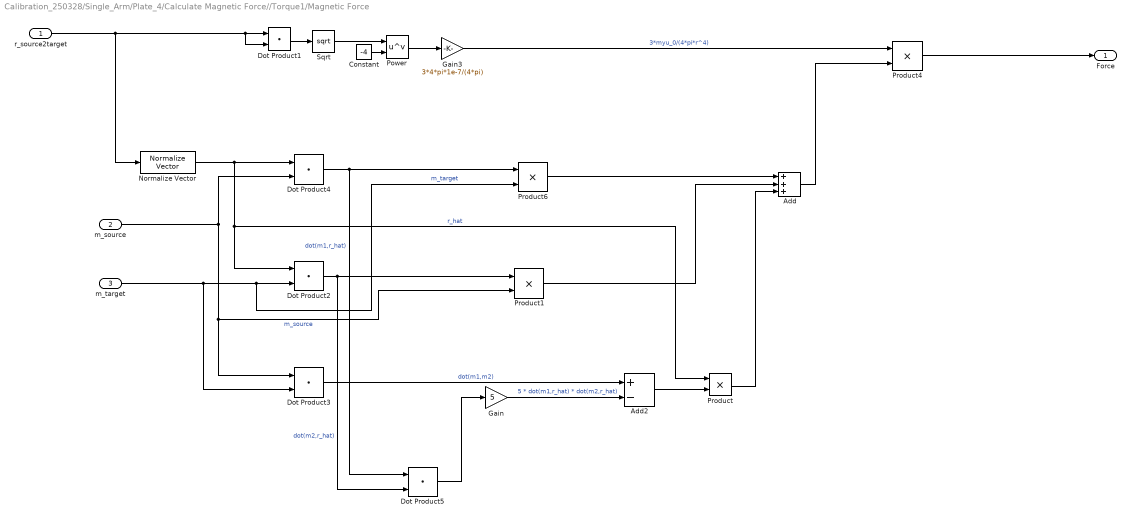
== system Calibration_250328/Single_Arm/Plate_4/Calculate Magnetic Force//Torque1/Magnetic Force ==
  r_source2target : Inport
  m_source : Inport  Port=2
  m_target : Inport  Port=3
  Add : Sum  Inputs=+++
  Add2 : Sum  Inputs=+-
  Constant : Constant  Value=-4
  Dot Product{1..5} (5 alike) : DotProduct  OutDataTypeStr=Inherit: Inherit via internal rule
  Gain : Gain  Gain=5
  Gain3 : Gain  Gain=3*4*pi*1e-7/(4*pi)
  Normalize Vector : vrlib/Utilities/Normalize Vector  maxzero=0
  Power : Math  Operator=pow
  Product{,1,4,6} (4 alike) : Product
  Sqrt : Sqrt
  Force : Outport
  wires:
  Dot Product1/1 -> Sqrt/1
  Constant/1 -> Power/2
  Power/1 -> Gain3/1
  Gain3/1 -> Product4/1  "3*myu_0/(4*pi*r^4)"
  Product4/1 -> Force/1
  r_source2target/1 -> Normalize Vector/1, Dot Product1/2, Dot Product1/1
  Normalize Vector/1 -> Product/1, Dot Product2/1, Dot Product4/1  "r_hat"
  m_source/1 -> Dot Product3/1, Product1/2, Dot Product4/2  "m_source"
  m_target/1 -> Dot Product3/2, Dot Product2/2, Product6/2  "m_target"
  Dot Product4/1 -> Product6/1, Dot Product5/1  "dot(m1,r_hat)"
  Dot Product2/1 -> Product1/1, Dot Product5/2  "dot(m2,r_hat)"
  Dot Product3/1 -> Add2/1  "dot(m1,m2)"
  Dot Product5/1 -> Gain/1
  Gain/1 -> Add2/2  "5 * dot(m1,r_hat) * dot(m2,r_hat)"
  Product1/1 -> Add/2
  Product6/1 -> Add/1
  Add/1 -> Product4/2
  Add2/1 -> Product/2
  Product/1 -> Add/3
  Sqrt/1 -> Power/1

== system Calibration_250328/Single_Arm/Plate_4/Calculate Magnetic Force//Torque1/Magnetic Torque ==
  note: 모든 좌표계는 World Frame 기준!
  r_source2target : Inport
  m_source : Inport  Port=2
  m_target : Inport  Port=3
  Add : Sum  Inputs=+-
  Constant : Constant  Value=-3
  Constant1 : Constant  Value=eye(3)
  Cross Product : matrix_library/Cross Product
  Dot Product : DotProduct  OutDataTypeStr=Inherit: Inherit via internal rule
  Gain : Gain  Gain=4*pi*1e-7/(4*pi)
  Gain1 : Gain  Gain=3
  MatrixMultiply : Product  Multiplication=Matrix(*)
  MatrixMultiply1 : Product  Multiplication=Matrix(*)
  Normalize Vector : vrlib/Utilities/Normalize Vector  maxzero=0
  Power : Math  Operator=pow
  Product : Product
  Sqrt : Sqrt
  Transpose : Math  Operator=transpose
  Torque : Outport
  wires:
  Cross Product/1 -> Torque/1
  m_target/1 -> Cross Product/1
  r_source2target/1 -> Dot Product/2, Dot Product/1, Normalize Vector/1
  Dot Product/1 -> Sqrt/1
  Constant/1 -> Power/2
  Power/1 -> Gain/1
  Normalize Vector/1 -> Transpose/1, MatrixMultiply/1
  Transpose/1 -> MatrixMultiply/2
  MatrixMultiply/1 -> Gain1/1
  Constant1/1 -> Add/2
  Add/1 -> MatrixMultiply1/1
  m_source/1 -> MatrixMultiply1/2
  Gain/1 -> Product/2
  MatrixMultiply1/1 -> Product/1
  Product/1 -> Cross Product/2
  Gain1/1 -> Add/1
  Sqrt/1 -> Power/1

== system Calibration_250328/Single_Arm/Plate_5/Calculate Magnetic Force//Torque1/Magnetic Force ==
  r_source2target : Inport
  m_source : Inport  Port=2
  m_target : Inport  Port=3
  Add : Sum  Inputs=+++
  Add2 : Sum  Inputs=+-
  Constant : Constant  Value=-4
  Dot Product{1..5} (5 alike) : DotProduct  OutDataTypeStr=Inherit: Inherit via internal rule
  Gain : Gain  Gain=5
  Gain3 : Gain  Gain=3*4*pi*1e-7/(4*pi)
  Normalize Vector : vrlib/Utilities/Normalize Vector  maxzero=0
  Power : Math  Operator=pow
  Product{,1,4,6} (4 alike) : Product
  Sqrt : Sqrt
  Force : Outport
  wires:
  Sqrt/1 -> Power/1
  Product/1 -> Add/3
  Add2/1 -> Product/2
  Add/1 -> Product4/2
  Product6/1 -> Add/1
  Product1/1 -> Add/2
  Gain/1 -> Add2/2  "5 * dot(m1,r_hat) * dot(m2,r_hat)"
  Dot Product5/1 -> Gain/1
  Dot Product3/1 -> Add2/1  "dot(m1,m2)"
  Dot Product2/1 -> Dot Product5/2, Product1/1  "dot(m2,r_hat)"
  Dot Product4/1 -> Dot Product5/1, Product6/1  "dot(m1,r_hat)"
  m_target/1 -> Product6/2, Dot Product2/2, Dot Product3/2  "m_target"
  m_source/1 -> Dot Product4/2, Product1/2, Dot Product3/1  "m_source"
  Normalize Vector/1 -> Dot Product4/1, Dot Product2/1, Product/1  "r_hat"
  r_source2target/1 -> Dot Product1/1, Dot Product1/2, Normalize Vector/1
  Product4/1 -> Force/1
  Gain3/1 -> Product4/1  "3*myu_0/(4*pi*r^4)"
  Power/1 -> Gain3/1
  Constant/1 -> Power/2
  Dot Product1/1 -> Sqrt/1

== system Calibration_250328/Single_Arm/Plate_5/Calculate Magnetic Force//Torque1/Magnetic Torque ==
  note: 모든 좌표계는 World Frame 기준!
  r_source2target : Inport
  m_source : Inport  Port=2
  m_target : Inport  Port=3
  Add : Sum  Inputs=+-
  Constant : Constant  Value=-3
  Constant1 : Constant  Value=eye(3)
  Cross Product : matrix_library/Cross Product
  Dot Product : DotProduct  OutDataTypeStr=Inherit: Inherit via internal rule
  Gain : Gain  Gain=4*pi*1e-7/(4*pi)
  Gain1 : Gain  Gain=3
  MatrixMultiply : Product  Multiplication=Matrix(*)
  MatrixMultiply1 : Product  Multiplication=Matrix(*)
  Normalize Vector : vrlib/Utilities/Normalize Vector  maxzero=0
  Power : Math  Operator=pow
  Product : Product
  Sqrt : Sqrt
  Transpose : Math  Operator=transpose
  Torque : Outport
  wires:
  Sqrt/1 -> Power/1
  Gain1/1 -> Add/1
  Product/1 -> Cross Product/2
  MatrixMultiply1/1 -> Product/1
  Gain/1 -> Product/2
  m_source/1 -> MatrixMultiply1/2
  Add/1 -> MatrixMultiply1/1
  Constant1/1 -> Add/2
  MatrixMultiply/1 -> Gain1/1
  Transpose/1 -> MatrixMultiply/2
  Normalize Vector/1 -> MatrixMultiply/1, Transpose/1
  Power/1 -> Gain/1
  Constant/1 -> Power/2
  Dot Product/1 -> Sqrt/1
  r_source2target/1 -> Normalize Vector/1, Dot Product/1, Dot Product/2
  m_target/1 -> Cross Product/1
  Cross Product/1 -> Torque/1

== system Calibration_250328/Single_Arm/Plate_6/Calculate Magnetic Force//Torque1/Magnetic Force ==
  r_source2target : Inport
  m_source : Inport  Port=2
  m_target : Inport  Port=3
  Add : Sum  Inputs=+++
  Add2 : Sum  Inputs=+-
  Constant : Constant  Value=-4
  Dot Product{1..5} (5 alike) : DotProduct  OutDataTypeStr=Inherit: Inherit via internal rule
  Gain : Gain  Gain=5
  Gain3 : Gain  Gain=3*4*pi*1e-7/(4*pi)
  Normalize Vector : vrlib/Utilities/Normalize Vector  maxzero=0
  Power : Math  Operator=pow
  Product{,1,4,6} (4 alike) : Product
  Sqrt : Sqrt
  Force : Outport
  wires:
  Dot Product1/1 -> Sqrt/1
  Constant/1 -> Power/2
  Power/1 -> Gain3/1
  Gain3/1 -> Product4/1  "3*myu_0/(4*pi*r^4)"
  Product4/1 -> Force/1
  r_source2target/1 -> Normalize Vector/1, Dot Product1/2, Dot Product1/1
  Normalize Vector/1 -> Product/1, Dot Product2/1, Dot Product4/1  "r_hat"
  m_source/1 -> Dot Product3/1, Product1/2, Dot Product4/2  "m_source"
  m_target/1 -> Dot Product3/2, Dot Product2/2, Product6/2  "m_target"
  Dot Product4/1 -> Product6/1, Dot Product5/1  "dot(m1,r_hat)"
  Dot Product2/1 -> Product1/1, Dot Product5/2  "dot(m2,r_hat)"
  Dot Product3/1 -> Add2/1  "dot(m1,m2)"
  Dot Product5/1 -> Gain/1
  Gain/1 -> Add2/2  "5 * dot(m1,r_hat) * dot(m2,r_hat)"
  Product1/1 -> Add/2
  Product6/1 -> Add/1
  Add/1 -> Product4/2
  Add2/1 -> Product/2
  Product/1 -> Add/3
  Sqrt/1 -> Power/1

== system Calibration_250328/Single_Arm/Plate_6/Calculate Magnetic Force//Torque1/Magnetic Torque ==
  note: 모든 좌표계는 World Frame 기준!
  r_source2target : Inport
  m_source : Inport  Port=2
  m_target : Inport  Port=3
  Add : Sum  Inputs=+-
  Constant : Constant  Value=-3
  Constant1 : Constant  Value=eye(3)
  Cross Product : matrix_library/Cross Product
  Dot Product : DotProduct  OutDataTypeStr=Inherit: Inherit via internal rule
  Gain : Gain  Gain=4*pi*1e-7/(4*pi)
  Gain1 : Gain  Gain=3
  MatrixMultiply : Product  Multiplication=Matrix(*)
  MatrixMultiply1 : Product  Multiplication=Matrix(*)
  Normalize Vector : vrlib/Utilities/Normalize Vector  maxzero=0
  Power : Math  Operator=pow
  Product : Product
  Sqrt : Sqrt
  Transpose : Math  Operator=transpose
  Torque : Outport
  wires:
  Cross Product/1 -> Torque/1
  m_target/1 -> Cross Product/1
  r_source2target/1 -> Dot Product/2, Dot Product/1, Normalize Vector/1
  Dot Product/1 -> Sqrt/1
  Constant/1 -> Power/2
  Power/1 -> Gain/1
  Normalize Vector/1 -> Transpose/1, MatrixMultiply/1
  Transpose/1 -> MatrixMultiply/2
  MatrixMultiply/1 -> Gain1/1
  Constant1/1 -> Add/2
  Add/1 -> MatrixMultiply1/1
  m_source/1 -> MatrixMultiply1/2
  Gain/1 -> Product/2
  MatrixMultiply1/1 -> Product/1
  Product/1 -> Cross Product/2
  Gain1/1 -> Add/1
  Sqrt/1 -> Power/1
